simulink library "common_lib"  (R2021b)
settings: Solver=ode45  StartTime=0.0  StopTime=10.0  RelTol=1e-3
undefined symbols (not defined in the file or in its folder): ACCEL_PRE_MULT, C_C1GearNumbers, C_C1GearRatios, C_Calibration, C_DitherWaveform, C_GearOffset, C_GearRatioIn, C_GearRatioInverseOut, C_GearRatioOut, CLUTCH_INNER_LOOP_UPDATE_RATE, CONSTANT, DEGRADED_MODE_SIZE, Dem_EventStatusType, DiscIntNeverNeededParam, F_FAULT_ENUM, F_NOFAULT, F_OUTOFRANGE, F_RATELIMIT, FALSE, FMI14_SPECIAL_INSTRUCTIONS, FMI20_DATA_DRIFTED_HIGH, FMI21_DATA_DRIFTED_LOW, FMI29_RESERVED_FOR_SAE_ASSIGNMENT, FMI30_RESERVED_FOR_SAE_ASSIGNMENT, FMI31_CONDITION_EXISTS, FMI32_NO_FAULT, IC, k_accel, k_mean, LVDCU_OORH_FaultCntThd_C, MAX_UINT32, MEAN_PRE_MULT, NTriggers, QLTY_SIGNAL_FAILED, QLTY_SIGNAL_FULLY_FUNCTION, QLTY_SIGNAL_SUBSTITUTED_BY_1ST_CHOICE, QLTY_SIGNAL_SUBSTITUTED_BY_2ND_CHOICE, QLTY_SIGNAL_SUBSTITUTED_BY_3RD_CHOICE, QLTY_SIGNAL_SUBSTITUTED_BY_4TH_CHOICE, SAMPLE_TIME_100_mSec, SAMPLE_TIME_100_uSec, simin, T_TestPoint, TF_FALSE, TF_TRUE, TimeStep, TRUE, WORKSPACE_UPDATE_RATE, ZERO, Zero
libraries: $bdroot x120, simulink x27, simulink_extras x4, MBD_EPS_Local_Blockset x4
(part 3 of 10)

== system common_lib/SCond ==
  note: Signal Conditioning
  Gain and Offset (in) : Subsystem  mask(CL Gain And Offset (in)){DataType=Single}
      mask prompts: DataType "Output Data Type"
      mask help:
      | Gain/Offset with data type coercion
      |
      | NgEK, Inc.
      mask init:
      | h=gcb;
      | 
      | set_param([h '/InputConversion'], 'DataType','single');
      | set_param([h '/InputConversion1'], 'DataType','single');
      | set_param([h '/InputConversion2'], 'DataType','single');
      | 
      | switch DataType
      |   case (1)
      |       set_param([h '/OutputConversion'], 'DataType','int8');
      |  case (2)
      |       set_param([h '/OutputConversion'], 'DataType','uint8');
      |    case (3)
      |       set_param([h '/OutputConversion'], 'DataType','int16');
      |  case (4)
      |      set_param([h '/OutputConversion'], 'DataType','uint16');
      |   case (5)
      |         set_param([h '/OutputConversion'], 'DataType','single');
      |    case (6)
      |         set_param([h '/InputConversion'], 'DataType','double');
      |         set_param([h '/InputConversion1'], 'DataType','double');
      |         set_param([h '/InputConversion2'], 'DataType','double');
      |      set_param([h '/OutputConversion'], 'DataType','double');    
      |    otherwise
      |      set_param([h '/OutputConversion'], 'DataType','single');
      | end
      mask Help: web(which(['common_lib32.html']))
      mask TypeOptions DataType: Int8 | UInt8 | Int16 | UInt16 | Single | Double
      mask Display:
      | patch([0.35 0.35 0.65 0.65], [0.35 0.65 0.65 0.35], [255/255 127/255 255/255]);
      | disp(['mx-b']);
  Gain and Offset (out) : Subsystem  mask(CL Gain And Offset (out)){DataType=Single}
      mask prompts: DataType "Output Data Type"
      mask help:
      | Gain/Offset with data type coercion
      |
      | NgEK, Inc.
      mask init: same as common_lib/SCond/Gain and Offset (in)
      mask Help: web(which(['common_lib33.html']))
      mask TypeOptions DataType: Int8 | UInt8 | Int16 | UInt16 | Single | Double
      mask Display:
      | patch([0.35 0.35 0.65 0.65], [0.35 0.65 0.65 0.35], [255/255 127/255 255/255]);
      | disp(['(x+b)/m']);
  Membership Function : Subsystem  mask(CL Membership Function){Low=single(10), Peak=single(50), High=single(90), DType=Upper Trapezoid}
      mask prompts: Low "Lower Value"; Peak "Peak Value"; High "Upper Value"; DType "Membership Type"
      mask help:
      | Triangular membership function calculation with an output of 1 at the "Peak" value and dropping off to 0 towards the "Low" and "High" values.  End "trapezoid" membership functions may be specified with the membership "type" pulldown menu.
      |
      | X(1) = Independent Variable
      |
      | Y(1) = Membership Function (0:1)
      |
      | NgEK, Inc.
      mask init:
      | if Peak<Low | Peak>High, disp(['WARNING: Breakpoints Non-Monotonic in <' gcb '>!']), end
      | 
      | switch class(Peak)
      |   case ('double')
      |        Zero      = double( 0.0);
      |          One       = double( 1.0);
      |         if (DType==1)
      |             SlopeLow  = 0.0;
      |           SlopeHigh = 1.0/(Peak-High);
      |         elseif (DType==2)
      |             SlopeLow  = 1.0/(Peak-Low);
      |            SlopeHigh = 1.0/(Peak-High);
      |       else
      |          SlopeLow  = 1.0/(Peak-Low);
      |           SlopeHigh = 0.0;
      |        end;
      |      
      |     case ('single')
      |        Zero      = single( 0.0);
      |          One       = single( 1.0);
      |        if (DType==1)
      |            SlopeLow  = single(0.0);
      |           SlopeHigh = single(1.0/(double(Peak)-double(High)));
      |          elseif (DType==2)
      |            SlopeLow  = single(1.0/(double(Peak)-double(Low)));
      |            SlopeHigh = single(1.0/(double(Peak)-double(High)));
      |       else
      |          SlopeLow  = single(1.0/(double(Peak)-double(Low)));
      |           SlopeHigh = single(0.0);
      |         end;
      | end;
      | 
      | if     (abs(double(SlopeLow))<abs(double(SlopeHigh)))
      |   XPltAxis = [ 0 0.2 0.7 0.8 1.0 ];
      | elseif (abs(double(SlopeHigh))<abs(double(SlopeLow)))
      |  XPltAxis = [ 0 0.2 0.3 0.8 1.0 ];
      | else
      |  XPltAxis = [ 0 0.2 0.5 0.8 1.0 ];
      | end;
      | 
      | if     (DType==1)
      |        YPltAxis = [ 1 1 0 0 0 ];
      | elseif (DType==2)
      |        YPltAxis = [ 0 0 1 0 0 ];
      | else
      |        YPltAxis = [ 0 0 0 1 1 ];
      | end;
      mask Help: web(which(['common_lib36.html']))
      mask TypeOptions DType: Lower Trapezoid | Central Triangle | Upper Trapezoid
      mask Display:
      | patch([.2 .2 .8 .8],[.2 .85 .85 .2],[255/255 127/255 255/255])
      | plot(XPltAxis, YPltAxis);
      | disp(['Low=',num2str(double(Low)),sprintf('\n'),'Peak=',num2str(double(Peak)),sprintf('\n'),'High=',num2str(double(High))])
  Test Override Gain and Offset (in) : Subsystem  mask(CL Gain And Offset (in)){DataType=Single}
      mask prompts: DataType "Output Data Type"
      mask help: Gain/Offset with enabled Gain and Offset option and with Output data type conversion
      mask init: same as common_lib/SCond/Gain and Offset (in)
      mask TypeOptions DataType: Int8 | UInt8 | Int16 | UInt16 | Single | Double
      mask Display:
      | patch([0.3 0.3 0.7 0.7], [0.35 0.65 0.65 0.35], [255/255 127/255 255/255])
      | disp(['Y=mX+b\nTest Override'])
  ramp to zero : Subsystem  mask(CL Ramp to Zero){DataType=Single}
      mask prompts: DataType "Data Type"
      mask help:
      | Ramp input signal to zero
      |
      | X(1) = Speed
      | X(2) = Limit
      |
      | Y(1) = Factor
      |
      | NgEK, Inc.
      mask init:
      | switch DataType
      |     case (1)
      |        One      = single( 1.0);
      |          MinusOne = single(-1.0);
      |         Zero     = single( 0.0);
      |     case (2)
      |         One      = double( 1.0);
      |          MinusOne = double(-1.0);
      |       Zero     = double( 0.0);
      | end;
      mask Help: web(which(['common_lib34.html']))
      mask TypeOptions DataType: Single | Double
      mask Display:
      | patch([0.3 0.3 0.7 0.7], [0.3 0.7 0.7 0.3], [255/255 127/255 255/255]);
      | disp('ramp to\nzero')

== system common_lib/Signal Conditioning ==
  note: Signal Conditioning
  2nd Order Butterworth Filter : Subsystem  mask{IC=0, TSAMP=0}
      mask prompts: IC "Initial Condition"; TSAMP "Sample Time"
      mask Display:
      | patch([0.35 0.35 0.65 0.65], [0.3 0.7 0.7 0.3], [255/255 127/255 255/255])
      | disp('2nd Order\nButterworth')
      | port_label('input',1,'input')
      | port_label('input',2,'cutoff_freq')
      | port_label('input',3,'reset')
      | port_label('output',1,'output')
  AnalogChecking : Subsystem  TreatAsAtomicUnit=on  mask{TimeStep=[]}
      mask prompts: TimeStep "Time Step"
  DitherSaturation : Subsystem  Description=|
      | This block generates dither using the table given for DitherWaveform at the frequency and amplitude given by the freq_hz and amplitude inputs.  All inputs should be 'single' datatype.  The table should be 'single' data type also.  The block runs at the sample time of the 'in' input.  It generates the correct frequency dither regardless of sample time.
      |                                                                                                                                                                                                                                                                                                                                                                  
      | Since it may not be possible to generate the exact frequency specified in the 'freq_hz' input, the block puts out the actual frequency in the 'realized_frequency' output.
  DitherSaturation1 : Subsystem  Description=|
      | This block generates dither using the table given for DitherWaveform at the frequency and amplitude given by the freq_hz and amplitude inputs.  All inputs should be 'single' datatype.  The table should be 'single' data type also.  The block runs at the sample time of the 'in' input.  It generates the correct frequency dither regardless of sample time.
      |                                                                                                                                                                                                                                                                                                                                                                  
      | Since it may not be possible to generate the exact frequency specified in the 'freq_hz' input, the block puts out the actual frequency in the 'realized_frequency' output.
  HydValveDither : Subsystem  Description=|  mask{DitherWaveform=single(C_DitherWaveform), ts=0}
      | This block generates dither using the table given for DitherWaveform at the frequency and amplitude given by the freq_hz and amplitude inputs.  All inputs should be 'single' datatype.  The table should be 'single' data type also.  The block runs at the sample time of the 'in' input.  It generates the correct frequency dither regardless of sample time.
      |                                                                                                                                                                                                                                                                                                                                                                  
      | Since it may not be possible to generate the exact frequency specified in the 'freq_hz' input, the block puts out the actual frequency in the 'realized_frequency' output.
      mask prompts: DitherWaveform "Dither Waveform"; ts "Sample Time"
  Normalized Variable Tanh Curve : Subsystem  mask{TimeStep=TimeStep}
      mask prompts: TimeStep "Sample Time"
      mask Display:
      | patch([0.3 0.3 0.7 0.7], [0.35 0.65 0.65 0.35], [255/255 127/255 255/255])
      | plot([0:.05:1],(tanh(([0:.05:1]*2*pi)-pi)+1)/2)
      | port_label('input',1,'RampTime')
      | port_label('input',2,'Reset')
      | port_label('output',1,'Out')
  Obsolete Signal Conditioning : Subsystem
      mask Display: disp('Obsolete\nSignal\nConditioning')
  OffsetAndGain : Subsystem  TreatAsAtomicUnit=on  mask(CL_OffsetAndGain){}
      mask help: Gain/Offset
      mask Help: web(which(['common_lib32.html']))
      mask Display:
      | patch([0.3 0.3 0.7 0.7], [0.4 0.6 0.6 0.4], [205/255 205/255 255/255]);
      | disp(['m*(x+b)']);
  SpeedProcess : Subsystem
  Trajectory : Subsystem  mask{TimeStep=TimeStep, wn=single(30), damping=single(.8)}
      mask prompts: TimeStep "Sample Time"; wn "Natural Frequency"
      mask Display:
      | patch([0.325 0.325 0.675 0.675], [0.35 0.65 0.65 0.35], [255/255 127/255 255/255])
      | disp('Trajectory')
      | port_label('input',1,'In')
      | port_label('input',2,'MaxAccel')
      | port_label('input',3,'MinAccel')
      | port_label('input',4,'MaxJerk')
      | port_label('input',5,'MinJerk')
      | port_label('input',6,'Reset')
      | port_label('output',1,'Out')
  Variable Tanh Curve : Subsystem  mask{TimeStep=TimeStep}
      mask prompts: TimeStep "Sample Time"
      mask Display:
      | patch([0.3 0.3 0.7 0.7], [0.35 0.65 0.65 0.35], [255/255 127/255 255/255])
      | plot([0:.05:1],(tanh(([0:.05:1]*2*pi)-pi)+1)/2)
      | port_label('input',1,'StartValue')
      | port_label('input',2,'FinalValue')
      | port_label('input',3,'RampTime')
      | port_label('input',4,'Reset')
      | port_label('output',1,'Out')
      | port_label('output',2,'RampComplete')

== system common_lib/Signal Generators ==
  note: Signal Generators
  Clu_2_1_3_1_1_1_TestSignalBuilder : Subsystem
  CustomProfileGenerator : Subsystem  mask{TimeStep=single(0.002)}
      mask prompts: TimeStep "Time Step"
  Signal Generator Components : Subsystem
      mask Display: disp('Signal\nGenerators\nComponents')
  SquareTriangleWaveDither : Subsystem  mask{TimeStep=single(0.002)}
      mask prompts: TimeStep "Time Step"
  SquareTriangleWaveDitherPWM : Subsystem  mask{TimeStep=single(0.002)}
      mask prompts: TimeStep "Time Step"
  SquareTriangleWaveGenerator_Advanced : Subsystem  mask{TimeStep=0}
      mask prompts: TimeStep "Time Step"
  SquareTriangleWaveGenerator_Basic : Subsystem  mask{TimeStep=0}
      mask prompts: TimeStep "Time Step"

== system common_lib/Signal Routing ==
  note: Signal Routing
  Overwrite : Subsystem  mask{VarName=VariableName, OverwriteEnable=off, OverwriteValue=0}
      mask prompts: VarName "Name"; OverwriteEnable "Overwrite ?"; OverwriteValue "Value"
      mask init:
      | enabled = strncmpi(get_param(gcb, 'OverwriteEnable'), 'on', 2);
      | 
      | if (enabled)
      |     dispname = char(get_param(gcb, 'OverwriteValue'));
      | else
      |     dispname = char('No Overwrite');
      | end
      | 
      | dispname = [VarName '\n' dispname];
      | 
      | %
      | % Change the name of the constants to match the VarName
      | %
      | rtblockname = char(find_system(gcb, 'LookUnderMasks', 'all', 'FollowLinks', 'on', 'BlockType', 'Constant'));
      | 
      | % The first constant should be the overwrite enable
      | set_param(deblank(rtblockname(1,:)), 'Name', strcat('xPCOE_', VarName));
      | 
      | % The second constant should be the overwrite value
      | set_param(deblank(rtblockname(2,:)), 'Name', strcat('xPCOV_', VarName));
      mask Display: disp(dispname)
  Vector to Bus : Subsystem  mask(Vector To Bus){BOName=BO_}
      mask prompts: BOName "Bus Object Name (Must be in workspace)"
      mask help:
      | This block takes in a vector and adds the signal names specified in the bus
      | object.  The output is a bus.
      |
      | In the present state of development this block only works for 8 input elements.
      mask init:
      | % Set the number of signals in the input mux.  This should really come from
      | % the dialog box. 
      | NumInputs = 8;
      | 
      | % Get the name of the bus object
      | BOName = get_param(gcb, 'BOName');
      | 
      | % If this workspace var is not of type Simulink.Bus there is a problem
      | a = evalin('base', ['whos(''' BOName ''')']);
      | 
      | if (length(a)==0) 
      |     error('The dialog must specify a valid Simulink.Bus')
      | end
      | if (strcmp(a.class, 'Simulink.Bus')==0)
      |     error('The dialog must specify a valid Simulink.Bus')
      | end
      | 
      | % Find the number of elements in the bus object
      | BONumelm = evalin('base', ['length(' BOName '.Elements)']);
      | 
      | % Get the names from the bus object
      | for x=1:BONumelm
      |     SigNames{x} = evalin('base', [BOName '.Elements(' sprintf('%i',x) ').Name']);
      | end
      | 
      | % Find the bus creator
      | BusCreator = char(find_system(gcb, 'LookUnderMasks', 'all', 'FollowLinks', 'on', 'BlockType', 'BusCreator'));
      | p = get_param(BusCreator, 'PortHandles');
      | l = get_param(p.Inport, 'Line');
      | 
      | % Assign the names to the signals going into the bus creator
      | for x=1:NumInputs
      |     if (x<=BONumelm)
      |        set_param(l{x}, 'Name', SigNames{x});
      |     else
      |        set_param(l{x}, 'Name', sprintf('Signal%i', x));
      |     end
      | end
      mask Display: disp(BOName)

== system common_lib/Slink ==
  note: Simulink Enhancements
  Dead : Subsystem  mask(CL Variable Deadband){DataType=Single}
      mask prompts: DataType "Data Type"
      mask help:
      | Deadband with smooth output transition from deadband region.
      |
      | X(1) = input
      | X(2) = deadband
      |
      | Y(1) = output
      | NgEK, Inc.
      mask init:
      | switch DataType
      |     case (1)
      |        Zero     = double( 0.0);
      |          MinusOne = double(-1.0);
      |     case (2)
      |          Zero     = single( 0.0);
      |       MinusOne = single(-1.0);
      |    case (3)
      |        Zero     = int8( 0.0);
      |         MinusOne = int8(-1.0);
      |     case (4)
      |        Zero     = int16( 0.0);
      |       MinusOne = int16(-1.0);
      |     case (5)
      |          Zero     = int32( 0.0);
      |          MinusOne = int32(-1.0);
      | end;
      mask Help: web(which(['common_lib35.html']))
      mask TypeOptions DataType: Double | Single | Int8 | Int16 | Int32
      mask Display:
      | patch([0.3 0.3 0.7 0.7], [0.35 0.65 0.65 0.35], [255/255 127/255 255/255])
      | 
      | plot([0 1],[0.5 0.5], [0.5 0.5],[0 1], [0.1 0.35],[0.1 0.5], [0.65 0.9],[0.5 0.9])
  Hysteresis : Subsystem  mask(CL Hysteresis){IC=[]}
      mask prompts: IC "Initial Condition"
      mask help:
      | Hysteresis block
      |
      | X(1) = Input
      | X(2) = Deadband Width
      |
      | Y(1) = Output
      | NgEK, Inc.
      mask init:
      | switch class(IC)
      |    case ('double')
      |         MinusOne = double(-1.0);
      |  case ('single')
      |        MinusOne = single(-1.0);
      |  case ('int8')
      |       MinusOne = int8(-1.0);
      |     case ('int16')
      |       MinusOne = int16(-1.0);
      |     case ('int32')
      |          MinusOne = int32(-1.0);
      | end;
      mask Help: web(which(['common_lib42.html']))
      mask Display:
      | patch([0.3 0.3 0.7 0.7], [0.35 0.65 0.65 0.35], [255/255 127/255 255/255])
      | 
      | plot([0 .6 .75 1],[.25 .25 .75 .75], [.25 .4 .75],[.25 .75 .75], [.4 .5 .4],[.35 .25 .15], [.6 .5 .6],[.85 .75 .65])
  Relay : Subsystem  mask(CL Relay){init=[]}
      mask prompts: init "Initiailization State"
      mask help:
      | Relay block
      |
      | X(1) = Input
      | X(2) = Upper Threshold
      | X(3) = Lower Threshold
      | X(4) = Upper Value
      | X(5) = Lower Value
      |
      | Y(1) = output
      | NgEK, Inc.
      mask Help: web(which(['common_lib41.html']))
      mask Display:
      | patch([0.3 0.3 0.7 0.7], [0.35 0.65 0.65 0.35], [255/255 127/255 255/255])
      | 
      | plot([0 .75 .75 1],[.25 .25 .75 .75], [.25 .25 .75],[.25 .75 .75], [.4 .5 .4],[.35 .25 .15], [.6 .5 .6],[.85 .75 .65])
  Relay_1 : Subsystem  mask(CL Relay){}
      mask help:
      | Relay block
      |
      | X(1) = Input
      | X(2) = hysterisis
      | X(3) = Ending Point
      | Y(1) = output
      | NgEK, Inc.
      mask Help: web(which(['common_lib41.html']))
      mask Display:
      | patch([0.3 0.3 0.7 0.7], [0.35 0.65 0.65 0.35], [255/255 127/255 255/255])
      | 
      | plot([0 .75 .75 1],[.25 .25 .75 .75], [.25 .25 .75],[.25 .75 .75], [.4 .5 .4],[.35 .25 .15])
      | 
      | port_label('input', 1, 'Input')
      | port_label('input', 2, 'dead band')
      | port_label('input', 3, 'B')
      | port_label('output', 1, 'out')
  Sat : Subsystem  mask(CL Variable Saturation){}
      mask help:
      | Variable saturation block
      |
      | X(1) = input
      | X(2) = upper limit
      | X(3) = lower limit
      |
      | Y(1) = output
      | NgEK, Inc.
      mask Help: web(which(['common_lib37.html']))
      mask Display:
      | patch([0.3 0.3 0.7 0.7], [0.35 0.65 0.65 0.35], [255/255 127/255 255/255])
      | 
      | plot([0 1],[0.5 0.5],[0.5 0.5],[0 1],[0 0.25 0.75 1],[0 0 1 1])
  Three Value Threshold : Subsystem  mask(CL ThreeValuedThreshold){}
      mask help:
      | Relay block
      |
      | X(1) = Input
      | X(2) = Upper Threshold
      | X(3) = Lower Threshold
      | X(4) = Upper Value
      | X(5) = Between Value
      | X(6) = Lower Value
      |
      | Y(1) = output
      | NgEK, Inc.
      mask Help:
      | Relay block
      | 
      | X(1) = Input
      | X(2) = Upper Threshold
      | X(3) = Lower Threshold
      | X(4) = Upper Value
      | X(5) = Between Value
      | X(6) = Lower Value
      | 
      | Y(1) = output
      | NgEK, Inc.
      mask Display:
      | patch([0.3 0.3 0.7 0.7], [0.35 0.65 0.65 0.35], [255/255 127/255 255/255])
      | 
      | plot([0 0.25 0.25 0.75 0.75 1],[0.25 0.25 0.5 0.5 0.75 0.75]);
      | 
      | %plot([0 .75 .75 1],[.25 .25 .75 .75], [.25 .25 .75],[.25 .75 .75], [.4 .5 .4],[.35 .25 .15], [.6 .5 .6],[.85 .75 .65])
  Variable Rate Limiter : Subsystem  mask(CL Variable Rate Limiter){TimeStep=, ic=}
      mask prompts: TimeStep "Time Step"; ic "Initial Condition"
      mask help:
      | Variable rate limiter block
      |
      | X(1) = input
      | X(2) = rise rate
      | X(3) = fall rate
      |
      | Y(1) = output
      | NgEK, Inc.
      mask Help: web(which(['common_lib38.html']))
      mask Display:
      | patch([0.3 0.3 0.7 0.7], [0.35 0.65 0.65 0.35], [255/255 127/255 255/255])
      | 
      | plot([0 1],[0.5 0.5],[0.5 0.5],[0 1],[0 1],[0 1],[0.7 0.8 0.8],[0.8 0.8 0.7], [0.2 0.2 0.3],[0.3 0.2 0.2])
  Variable Rate Limiter w IC : Subsystem  mask(CL Variable Rate Limiter with Initial Condition){TimeStep=, ic=}
      mask prompts: TimeStep "Time Step"; ic "Initial Condition"
      mask help:
      | Variable rate limiter block with Initial Condiiton
      |
      | X(1) = input
      | X(2) = rise rate
      | X(3) = fall rate
      | X(4) = initial condition
      | X(5) = reset?
      |
      | Y(1) = output
      | NgEK, Inc.
      mask Help: web(which(['common_lib39.html']))
      mask Display:
      | patch([0.3 0.3 0.7 0.7], [0.35 0.65 0.65 0.35], [255/255 127/255 255/255])
      | 
      | plot([0 1],[0.5 0.5],[0.5 0.5],[0 1],[0 1],[0 1],[0.7 0.8 0.8],[0.8 0.8 0.7], [0.2 0.2 0.3],[0.3 0.2 0.2])
  Variable Rate Limiter w IC and Sat : Subsystem  mask(CL Variable Rate Limiter with IC and Saturation){TimeStep=, ic=}
      mask prompts: TimeStep "Time Step"; ic "Initial Condition"
      mask help:
      | Variable rate limiter block with Initial Condition and Saturation
      |
      | X(1) = input
      | X(2) = rise rate
      | X(3) = fall rate
      | X(4) = upper limit
      | X(5) = lower limit
      | X(6) = initial condition
      | X(7) = reset?
      |
      | Y(1) = output
      | NgEK, Inc.
      mask Help: web(which(['common_lib40.html']))
      mask Display:
      | patch([0.3 0.3 0.7 0.7], [0.35 0.65 0.65 0.35], [255/255 127/255 255/255])
      | 
      | plot([0 1],[0.5 0.5],[0.5 0.5],[0 1],[0 0.25 0.75 1],[0 0 1 1],[0.3 0.3 0.45],[0.25 0.1 0.2],[0.55 0.7 0.75],[0.8 0.9 0.78])

== system common_lib/Tbl ==
  note: Tables
  2D Lookup : Subsystem  TreatAsAtomicUnit=on  RTWFcnName=VARTABLE  mask(CL 2D Table Lookup){Mode=Linear Interpolation}
      mask prompts: Mode "Interpolation Mode"
      mask help:
      | 2D Table lookup with explicit axis inputs
      |
      | X(1) = Independent variable
      | X(2) = X axis vector
      | X(3) = Y axis vector
      |
      | Y(1) = output
      |
      | Interpolation mode is selected via the mask:
      |
      | Ceiling Interpolation: rounds up in the positive direction
      | Floor Interpolation: rounds down in the negative direction
      | Nearest (Neighbor) Interpolation: rounds to the closest representable number
      | Linear Interpolation: Interpolates data by assuming data varies linearly between points
      |
      | NgEK, Inc.
      settings: RTWFcnNameOpts=User specified  RTWFileNameOpts=Use function name
      mask Help: web(which(['common_lib45.html']))
      mask TypeOptions Mode: Linear Interpolation | Nearest Neighbor | Floor | Ceiling
      mask Display:
      | patch([0.3 0.3 0.7 0.7], [0.35 0.65 0.65 0.35], [255/255 127/255 255/255])
      | 
      | plot([0.2 0.2],[0.2 0.8],[0.2 0.8],[0.2 0.2],linspace(0.2,0.8,10),0.2+0.8*linspace(0.2,0.8,10).^2)
  Direct Look-Up Table (n-D) : LookupNDDirect
      settings: AttributesFormatString=%<mxTable>
  Interpolator : Subsystem  mask(CL Interpolation){DType=Double}
      mask prompts: DType "Data Type"
      mask help:
      | 1D Interpolation Block
      |
      | X(1) = value at 1
      | X(2) = value at 0
      | X(3) = interpolation value
      |
      | Y(1) = output
      | NgEK, Inc.
      mask init:
      | switch DType
      |    case (1)
      |       set_param([gcb '/XY Interpolator'],'DType','double');
      |        Zero = double(0.0);
      |          One  = double(1.0);
      |     case (2)
      |        set_param([gcb '/XY Interpolator'],'DType','single');
      |         Zero = single(0.0);
      |        One  = single(1.0);
      | end;
      mask Help: web(which(['common_lib43.html']))
      mask TypeOptions DType: Double | Single
      mask Display:
      | patch([0.3 0.3 0.7 0.7], [0.35 0.65 0.65 0.35], [255/255 127/255 255/255])
      | 
      | plot([.2 .9],[0.5 0.5],[0.2 0.3 0.8 .9],[.25 .25 .75 .75])
      | 
      | port_label('input', 1, '1')
      | port_label('input', 2, '0')
      | port_label('input', 3, 'interp')
  Look-Up Table : Lookup  InputValues=[-5:5]  Table=tanh([-5:5])  LookUpMeth=Interpolation-Use End Values
      settings: AttributesFormatString=%<OutputValues>
  Look-Up Table (2-D) : Lookup2D  RowIndex=[1:3]  ColumnIndex=[1:3]  Table=[4 5 6;16 19 20;10 18 23]  LookUpMeth=Interpolation-Use End Values
      settings: AttributesFormatString=%<OutputValues>
  XY Interpolator : Subsystem  TreatAsAtomicUnit=on  RTWFcnName=XYINT  mask(CL XY Interpolation){DType=single}
      mask prompts: DType "Data Type"
      mask help:
      | 2D Interpolation Block
      |
      | X(1) = output value at 1
      | X(2) = output value at 0
      | X(3) = input value corresponding to 1
      | X(4) = input value corresponding to 0
      | X(5) = input value
      |
      | Y(1) = output
      | NgEK, Inc.
      mask init:
      | switch DType
      |    case (1)
      |       set_param([gcb '/Interp'],...
      |          'FunctionName','xyinterp_f64_wrap',...
      |           'SFunctionModules','xyinterp_f64');
      | %        Zero = double(0.0);
      | %          One  = double(1.0);
      | %        Tol  = double(1e-6);
      |     case (2)
      |        set_param([gcb '/Interp'],...
      |           'FunctionName','xyinterp_f32_wrap',...
      |           'SFunctionModules','xyinterp_f32');
      | %        Zero = single(0.0);
      | %        One  = single(1.0);
      | %         Tol  = single(1e-6);
      | end;
      | % strDType = get_param(gcb,'DType');
      | % set_param([gcb '/DTC'],'OutDataTypeStr',strDType);
      | % set_param([gcb '/DTC1'],'OutDataTypeStr',strDType);
      | % set_param([gcb '/DTC2'],'OutDataTypeStr',strDType);
      | % set_param([gcb '/DTC3'],'OutDataTypeStr',strDType);
      | % set_param([gcb '/DTC4'],'OutDataTypeStr',strDType);
      settings: RTWFcnNameOpts=User specified  RTWFileNameOpts=Use function name
      mask Help: web(which(['common_lib44.html']))
      mask TypeOptions DType: double | single
      mask Display:
      | patch([0.3 0.3 0.7 0.7], [0.35 0.65 0.65 0.35], [255/255 127/255 255/255])
      | 
      | plot([.2 .9],[0.5 0.5],[0.2 0.3 0.8 .9],[.25 .25 .75 .75])
      | 
      | port_label('input', 1, 'Y_1')
      | port_label('input', 2, 'Y_0')
      | port_label('input', 3, 'X_1')
      | port_label('input', 4, 'X_0')
      | port_label('input', 5, 'X')
  XY Interpolator1 : Subsystem  TreatAsAtomicUnit=on  RTWFcnName=XYINT  mask(CL XY Interpolation){DType=single}
      mask prompts: DType "Data Type"
      mask help:
      | 2D Interpolation Block
      |
      | X(1) = output value at 1
      | X(2) = output value at 0
      | X(3) = input value corresponding to 1
      | X(4) = input value corresponding to 0
      | X(5) = input value
      |
      | Y(1) = output
      | NgEK, Inc.
      mask init:
      | switch DType
      |    case (1)
      |        Zero = double(0.0);
      |          One  = double(1.0);
      |        Tol  = double(1e-6);
      |     case (2)
      |        Zero = single(0.0);
      |        One  = single(1.0);
      |         Tol  = single(1e-6);
      | end;
      | strDType = get_param(gcb,'DType');
      | set_param([gcb '/DTC'],'OutDataTypeStr',strDType);
      | set_param([gcb '/DTC1'],'OutDataTypeStr',strDType);
      | set_param([gcb '/DTC2'],'OutDataTypeStr',strDType);
      | set_param([gcb '/DTC3'],'OutDataTypeStr',strDType);
      | set_param([gcb '/DTC4'],'OutDataTypeStr',strDType);
      settings: RTWSystemCode=Inline  RTWFcnNameOpts=User specified  RTWFileNameOpts=Use function name
      mask Help: web(which(['common_lib44.html']))
      mask TypeOptions DType: double | single
      mask Display:
      | patch([0.3 0.3 0.7 0.7], [0.35 0.65 0.65 0.35], [255/255 127/255 255/255])
      | 
      | plot([.2 .9],[0.5 0.5],[0.2 0.3 0.8 .9],[.25 .25 .75 .75])
      | 
      | port_label('input', 1, 'Y_1')
      | port_label('input', 2, 'Y_0')
      | port_label('input', 3, 'X_1')
      | port_label('input', 4, 'X_0')
      | port_label('input', 5, 'X')

== system common_lib/Timers ==
  note: Timers
  Timer : Subsystem  mask{TimeStep=0}
      mask prompts: TimeStep "Time Step (double)"
      mask help:
      | This block outputs a boolean true when In has been true
      | for at least the TiggerTime time.

== system common_lib/Approved Simulink/Basic IO ==
  note: HWin/ HWout
  note: Product Test
  note: Data Monitor, VPA, SnapShot
  Inport : Inport
  C_Calibration : $bdroot/IO/Calibration with Pretty Print Value  CalValue=C_Calibration  scaling=None
  Constant : Constant  Value=CONSTANT  SampleTime=-1
  DRDataStoreRead : DataStoreRead  DataStoreName=DataStoreRead  SampleTime=0  IndexOptions=Index vector (dialog)  Indices=1  OutputSizes=1
  DRDataStoreRead1 : DataStoreRead  DataStoreName=PT_ProductTest_Read  SampleTime=0  IndexOptions=Index vector (dialog)  Indices=1  OutputSizes=1
  DRDataStoreRead2 : DataStoreRead  DataStoreName=DM_DataMonitor_Read  SampleTime=0  IndexOptions=Index vector (dialog)  Indices=1  OutputSizes=1
  DSDataStoreMemory : DataStoreMemory  DataStoreName=DataStoreMemory  ShowAdditionalParam=off
  DSDataStoreMemory1 : DataStoreMemory  DataStoreName=PT_ProductTest_Memory  ShowAdditionalParam=off
  DSDataStoreMemory2 : DataStoreMemory  DataStoreName=DM_DataMonitor  ShowAdditionalParam=off
  DWDataStoreWrite : DataStoreWrite  DataStoreName=DataStoreWrite  IndexOptions=Index vector (dialog)  Indices=1  OutputSizes=1
  DWDataStoreWrite1 : DataStoreWrite  DataStoreName=DataStoreWrite  IndexOptions=Index vector (dialog)  Indices=1  OutputSizes=1
  DWDataStoreWrite2 : DataStoreWrite  DataStoreName=DM_DataMonitor_Write  IndexOptions=Index vector (dialog)  Indices=1  OutputSizes=1
  Ground : Ground
  M_MonitorParameter : ToWorkspace  VariableName=MonitorParameter  SampleTime=WORKSPACE_UPDATE_RATE
      settings: Decimation=WORKSPACE_DECIMATION
  M_MonitorParameter1 : Subsystem  mask{work=ToWorkspace}
      mask prompts: work "Variable Name"
      mask init:
      | set_param([gcb,'/towork'],'VariableName',work);
      | a = get_param([gcb '/Input'],'LineHandles');
      | set(a.Outport,'Name',work)
      mask Display:
      | patch([.01 .01 .99 .99],[.01 .99 .99 .01],[0 .8 0])
      | disp(work)
  T_TestPoint : Constant  Value=T_TestPoint  SampleTime=-1
  Terminator : Terminator
  To xPC Scope1 : Subsystem  mask(To Workspace Simulation){UserName=, SampleRate=-1, Prio=Low, NameFromSignal=on}
      mask prompts: UserName "Name"; SampleRate "Sample Rate"; Prio "Priority"; NameFromSignal "Name From Signal"
      mask help:
      | "Green Blocks" will record signals during simulation. The Name is now
      | required to come from the signal name so the "Name From Signal" box should
      | be checked. Please select the appropriate Priority Level to ensure optimal
      | simulation runtime and resource use.
      |
      | High - Will ALWAYS record. Choose this if it is a critical signal that
      |        everyone would benefit from having.
      |
      | Med  - A signal that is important to a particular subsystem for testing
      |        purposes. If testing that subsystem you will likely desire this
      |        signal
      |
      | Low  - For debug purposes within a subsystem. This is for obtaining maximum
      |        information in a subsystem to understand every step of logic during
      |        simulation
      mask init:
      | myPrio = 0;
      | sigName = '';
      | 
      | switch (Prio)
      |     case 'Low'
      |         myPrio = 3;
      |     case 'Med'
      |         myPrio = 2;
      |     case 'High'
      |         myPrio = 1;
      | end
      | 
      | if NameFromSignal || isempty(UserName)
      |     sigName = get_param(gcb, 'InputSignalNames');   % Get the name of the signal
      |     sigName = regexprep(sigName{1}, '[<> ]', '');
      | else
      |     sigName = UserName;
      | end
      | 
      | if ~isempty(sigName)
      |     if myPrio <= getPriority(char(gcb))
      |         tmLst = find_system(gcb, 'FollowLinks', 'on', 'LookUnderMasks', 'on', 'BlockType', 'Terminator');
      |         if ~isempty(tmLst)
      |             pos = get_param(tmLst{1}, 'Position');
      |             delete_block(tmLst{1});
      |             newPos = [pos(1), pos(2), pos(1) + 85, pos(2) + 20];
      |             add_block('built-in/ToWorkspace', [char(gcb) '/ToWorkspace'], ...
      |                 'Position', newPos, ...
      |                 'VariableName', ['SIMOUT_' char(sigName)], ...
      |                 'SampleTime', '-1', ...
      |                 'SaveFormat', 'Structure With Time', ...
      |                 'MaxDataPoints', 'Inf');
      |         end
      |     else
      |         twsLst = find_system(gcb, 'FollowLinks', 'on', 'LookUnderMasks', 'on', 'BlockType', 'ToWorkspace');
      |         if ~isempty(twsLst)
      |             pos = get_param(twsLst{1}, 'Position');
      |             delete_block(twsLst{1});
      |             newPos = [pos(1), pos(2), pos(1) + 20, pos(2) + 20];
      |             add_block('built-in/Terminator', [char(gcb) '/Terminate'], 'Position', newPos);
      |         end
      |     end
      | end
      mask TypeOptions Prio: Low | Med | High
      mask Display: disp(Prio)
  Outport : Outport  VectorParamsAs1DForOutWhenUnconnected=off

== system common_lib/Approved Simulink/Discrete And Discontinuities ==
  Dead Zone Dynamic : simulink/Discontinuities/Dead Zone Dynamic
      settings: SourceProductBaseCode=SL
  Discrete-Time Integrator : DiscreteIntegrator  ICPrevOutput=DiscIntNeverNeededParam  ICPrevScaledInput=DiscIntNeverNeededParam
  Rate Limiter : RateLimiter  SampleTimeMode=inherited
  Relay : Relay
  Saturation : Saturate
  Saturation Dynamic : simulink/Discontinuities/Saturation Dynamic  OutMin=[]  OutMax=[]  OutDataTypeStr=Inherit: Same as second input  OutDataType=fixdt(1, 16)  OutScaling=2^-10  DoSatur=off
  Unit Delay : UnitDelay  InitialCondition=IC  SampleTime=-1  HasFrameUpgradeWarning=on
      settings: AttributesFormatString=ic=%<X0>
  Zero-Order Hold : ZeroOrderHold

== system common_lib/Approved Simulink/Flip Flops ==
  D Flip-Flop : simulink_extras/Flip Flops/D Flip-Flop
  D Latch : simulink_extras/Flip Flops/D Latch
      settings: SourceProductBaseCode=SL
  J-K Flip-Flop : simulink_extras/Flip Flops/J-K Flip-Flop  initial_condition=0
  S-R Flip-Flop : simulink_extras/Flip Flops/S-R Flip-Flop  initial_condition=0

== system common_lib/Approved Simulink/Grouping ==
  note: Busses are preferred to
      | MUXes except where array definition
      | or linear algebra requires a MUX
  Bus Creator : BusCreator  Inputs=2
  Bus Selector : BusSelector  OutputSignals=signal1,signal2
  Demux : Demux  Outputs=2
  Merge : Merge
  Mux : Mux  Inputs=2
  Selector : Selector  InputPortWidth=3  IndexOptions=Index vector (dialog)  Indices=[1 3]  OutputSizes=1

== system common_lib/Approved Simulink/Math And Logic ==
  Abs : Abs  ZeroCross=off
  Assignment : Assignment  IndexOptions=Index vector (dialog)  Indices=1  OutputSizes=1
  Gain : Gain
  Logical Operator : Logic  Operator=OR  AllPortsSameDT=off
  Math Function : Math  SignedPower=on  SaturateOnIntegerOverflow=on
  MinMax : MinMax  Inputs=2  InputSameDT=on  ZeroCross=off
  Multiport Switch : MultiPortSwitch
  Product1 : Product  OutDataTypeStr=Inherit: Same as first input
  Relational Operator : RelationalOperator  Operator=<=  ZeroCross=off  RndMeth=Nearest
  Sign : Signum
  Sum : Sum  Inputs=|+-
  Switch : Switch  Threshold=0.5  ZeroCross=off

== system common_lib/Approved Simulink/Signal Attributes ==
  Data Type Conversion : DataTypeConversion  RndMeth=Zero
  Rate Transition : RateTransition
  Signal Conversion : SignalConversion  ConversionOutput=Contiguous copy  OverrideOpt=off

== system common_lib/Approved Simulink/SubSys Triggers ==
  Enable : EnablePort  ZeroCross=off
  Trigger : TriggerPort  VariantControl=(inherit)  ZeroCross=off
  Configurable Subsystem : Subsystem
      settings: TemplateBlock=self
  For Iterator Subsystem : Subsystem  TreatAsAtomicUnit=on
  Function-Call Generator : simulink/Ports & Subsystems/Function-Call Generator  sample_time=1  numberOfIterations=1  DisallowWideOutput=off
  If : If
  If Action Subsystem : Subsystem  TreatAsAtomicUnit=on
  Subsystem : Subsystem
  Switch Case : SwitchCase
  While Iterator Subsystem : Subsystem  TreatAsAtomicUnit=on

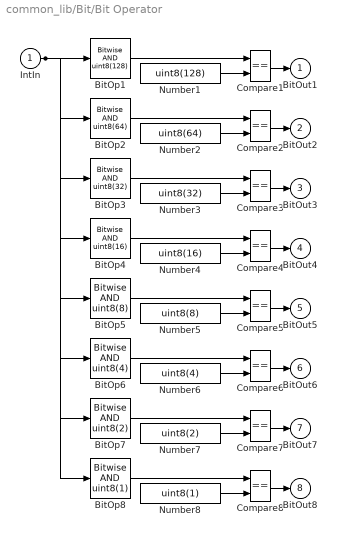
== system common_lib/Bit/Bit Operator ==
  IntIn : Inport
  BitOp1 : simulink/Logic and Bit Operations/Bitwise Operator  logicop=AND  UseBitMask=on  BitMask=uint8(128)  BitMaskRealWorld=Stored Integer
  BitOp2 : simulink/Logic and Bit Operations/Bitwise Operator  logicop=AND  UseBitMask=on  BitMask=uint8(64)  BitMaskRealWorld=Stored Integer
  BitOp3 : simulink/Logic and Bit Operations/Bitwise Operator  logicop=AND  UseBitMask=on  BitMask=uint8(32)  BitMaskRealWorld=Stored Integer
  BitOp4 : simulink/Logic and Bit Operations/Bitwise Operator  logicop=AND  UseBitMask=on  BitMask=uint8(16)  BitMaskRealWorld=Stored Integer
  BitOp5 : simulink/Logic and Bit Operations/Bitwise Operator  logicop=AND  UseBitMask=on  BitMask=uint8(8)  BitMaskRealWorld=Stored Integer
  BitOp6 : simulink/Logic and Bit Operations/Bitwise Operator  logicop=AND  UseBitMask=on  BitMask=uint8(4)  BitMaskRealWorld=Stored Integer
  BitOp7 : simulink/Logic and Bit Operations/Bitwise Operator  logicop=AND  UseBitMask=on  BitMask=uint8(2)  BitMaskRealWorld=Stored Integer
  BitOp8 : simulink/Logic and Bit Operations/Bitwise Operator  logicop=AND  UseBitMask=on  BitMask=uint8(1)  BitMaskRealWorld=Stored Integer
  Compare{1..8} (8 alike) : RelationalOperator  Operator===  RndMeth=Nearest  InputSameDT=on
  Number1 : Constant  Value=uint8(128)
  Number2 : Constant  Value=uint8(64)
  Number3 : Constant  Value=uint8(32)
  Number4 : Constant  Value=uint8(16)
  Number5 : Constant  Value=uint8(8)
  Number6 : Constant  Value=uint8(4)
  Number7 : Constant  Value=uint8(2)
  Number8 : Constant  Value=uint8(1)
  BitOut1 : Outport  VectorParamsAs1DForOutWhenUnconnected=off
  BitOut2 : Outport  Port=2  VectorParamsAs1DForOutWhenUnconnected=off
  BitOut3 : Outport  Port=3  VectorParamsAs1DForOutWhenUnconnected=off
  BitOut4 : Outport  Port=4  VectorParamsAs1DForOutWhenUnconnected=off
  BitOut5 : Outport  Port=5  VectorParamsAs1DForOutWhenUnconnected=off
  BitOut6 : Outport  Port=6  VectorParamsAs1DForOutWhenUnconnected=off
  BitOut7 : Outport  Port=7  VectorParamsAs1DForOutWhenUnconnected=off
  BitOut8 : Outport  Port=8  VectorParamsAs1DForOutWhenUnconnected=off
  wires:
  BitOp1/1 -> Compare1/1
  Number1/1 -> Compare1/2
  Compare1/1 -> BitOut1/1
  IntIn/1 -> BitOp1/1, BitOp2/1, BitOp3/1, BitOp4/1, BitOp5/1, BitOp6/1, BitOp7/1, BitOp8/1
  BitOp2/1 -> Compare2/1
  Number2/1 -> Compare2/2
  Compare2/1 -> BitOut2/1
  BitOp3/1 -> Compare3/1
  Number3/1 -> Compare3/2
  Compare3/1 -> BitOut3/1
  BitOp4/1 -> Compare4/1
  Number4/1 -> Compare4/2
  Compare4/1 -> BitOut4/1
  BitOp5/1 -> Compare5/1
  Number5/1 -> Compare5/2
  Compare5/1 -> BitOut5/1
  BitOp6/1 -> Compare6/1
  Number6/1 -> Compare6/2
  Compare6/1 -> BitOut6/1
  BitOp7/1 -> Compare7/1
  Number7/1 -> Compare7/2
  Compare7/1 -> BitOut7/1
  BitOp8/1 -> Compare8/1
  Number8/1 -> Compare8/2
  Compare8/1 -> BitOut8/1

== system common_lib/Ctrl/DTNA_PIgov ==
  note: During reset, integrator is set to zero
  note: Output - Pterm - Dterm = Iterm for saturation purposes
  note: Detect output saturation
  note: Common Library::Control Structures::PI Governor
  note: pterm
      | limited to output saturation limits
  error : Inport
  p_gain : Inport  Port=2
  i_gain : Inport  Port=3
  ulim : Inport  Port=4
  llim : Inport  Port=5
  reset? : Inport  Port=6  OutDataTypeStr=boolean
  Abs : Abs  ZeroCross=off  OutDataTypeStr=Inherit: Inherit via back propagation
  Constant1 : Constant  Value=MinInt  OutDataTypeStr=Inherit: Inherit via back propagation
  Constant2 : Constant  Value=MaxInt  OutDataTypeStr=Inherit: Inherit via back propagation
  Constant3 : Constant  Value=Zero
  Constant4 : Constant  Value=Zero
  Constant5 : Constant  Value=Tol  OutDataTypeStr=Inherit: Inherit via back propagation
  Integrator : Subsystem  TreatAsAtomicUnit=on  RTWFcnName=INTEGRATOR  mask(CL Integrator){TimeStep=TimeStep, IC=IC}
      mask prompts: TimeStep "Time Step"; IC "Initial Condition"
      mask help:
      | Determine the integral of the input.
      | If reset is true (1), the integrator is set to the reset condition input.
      |
      | X(1) = input
      | X(2) = upper limit
      | X(3) = lower limit
      | X(4) = reset condition
      | X(5) = reset
      |
      | Y(1) = output
      |
      | Time step is entered via mask parameter.
      | Initial condition is entered via mask parameter.
      |
      | NgEK, Inc.
      settings: RTWFcnNameOpts=User specified  RTWFileNameOpts=Use function name
      mask Help: web(which(['common_lib3.html']))
      mask Display:
      | patch([0.3 0.3 0.7 0.7], [0.35 0.65 0.65 0.35], [255/255 127/255 255/255])
      | disp('Integrator')
      | port_label('input', 1, 'input')
      | port_label('input', 2, 'ulim')
      | port_label('input', 3, 'llim')
      | port_label('input', 4, 'reset_cond')
      | port_label('input', 5, 'reset?')
      | port_label('output', 1, 'output')
  Logical Operator : Logic  Operator=OR
  Product1 : Product  InputSameDT=on  OutDataTypeStr=Inherit: Same as first input
  Product2 : Product  InputSameDT=on  OutDataTypeStr=Inherit: Same as first input
  Relational Operator : RelationalOperator  Operator=>  ZeroCross=off  RndMeth=Nearest  InputSameDT=on
  Sat : $bdroot/Slink/Sat
  Sat1 : $bdroot/Slink/Sat
  Sum1 : Sum  Inputs=+-  InputSameDT=on  OutDataTypeStr=Inherit: Same as first input
  Sum2 : Sum  Inputs=+-|  InputSameDT=on  OutDataTypeStr=Inherit: Same as first input
  Sum3 : Sum  InputSameDT=on  OutDataTypeStr=Inherit: Same as first input
  Switch : Switch  Threshold=0.5  ZeroCross=off  InputSameDT=on
  Switch1 : Switch  Threshold=0.5  ZeroCross=off  InputSameDT=on
  Unit Delay1 : UnitDelay  InitialCondition=Zero  SampleTime=-1  HasFrameUpgradeWarning=on
      settings: AttributesFormatString=ic=%<X0>
  Unit Delay2 : UnitDelay  InitialCondition=false  SampleTime=-1  HasFrameUpgradeWarning=on
      settings: AttributesFormatString=ic=%<X0>
  output : Outport  InitialOutput=8.973  VectorParamsAs1DForOutWhenUnconnected=off
  wires:
  Product2/1 -> Integrator/1(input)
  Sum1/1 -> Unit Delay1/1
  Integrator/1(Output) -> Sum3/2
  Switch/1 -> Integrator/4(ic)
  Unit Delay2/1 -> Logical Operator/2
  Logical Operator/1 -> Integrator/5(reset?)
  Constant4/1 -> Switch/1
  i_gain/1 -> Product2/2
  Sat/1 -> Sum2/2, output/1, Sum1/1
  Sum3/1 -> Sum2/1, Sat/1  "Actuator Signal"
  llim/1 -> Sat/3, Sat1/3
  Product1/1 -> Sat1/1, Sum3/1
  p_gain/1 -> Product1/1
  ulim/1 -> Sat/2, Sat1/2
  reset?/1 -> Switch/2, Switch1/2, Logical Operator/1
  Constant1/1 -> Integrator/3(llim)
  Constant2/1 -> Integrator/2(ulim)
  Constant5/1 -> Relational Operator/2
  Abs/1 -> Relational Operator/1
  Relational Operator/1 -> Unit Delay2/1
  Sum2/1 -> Abs/1
  Unit Delay1/1 -> Switch/3
  Sat1/1 -> Sum1/2
  Constant3/1 -> Switch1/1
  error/1 -> Switch1/3
  Switch1/1 -> Product2/1, Product1/2

== system common_lib/Ctrl/Derivative ==
  note: Common Library::Derivative
  input : Inport
  cutoff : Inport  Port=2
  ulim : Inport  Port=3
  llim : Inport  Port=4
  reset? : Inport  Port=5  OutDataTypeStr=boolean
  Data Type Conversion : DataTypeConversion  OutDataTypeStr=boolean
  Data Type Conversion1 : DataTypeConversion  OutDataTypeStr=single
  Data Type Conversion2 : DataTypeConversion  OutDataTypeStr=single
  DerivativeCoreLogic : Subsystem  TreatAsAtomicUnit=on  RTWFcnName=DER
      settings: RTWFcnNameOpts=User specified  RTWFileNameOpts=Use function name
  Gain : Gain  Gain=Ts
  Product1 : Product  Inputs=**  InputSameDT=on  OutDataTypeStr=Inherit: Same as first input
  Signal Conversion : SignalConversion  ConversionOutput=Contiguous copy  OverrideOpt=off
  output : Outport  VectorParamsAs1DForOutWhenUnconnected=off
  wires:
  input/1 -> Product1/1
  cutoff/1 -> Product1/2, Gain/1
  DerivativeCoreLogic/1(output) -> Signal Conversion/1
  reset?/1 -> Data Type Conversion/1
  Gain/1 -> DerivativeCoreLogic/2(cutoff)
  Product1/1 -> DerivativeCoreLogic/1(input)
  ulim/1 -> Data Type Conversion1/1
  llim/1 -> Data Type Conversion2/1
  Data Type Conversion/1 -> DerivativeCoreLogic/3(reset?)
  Data Type Conversion1/1 -> DerivativeCoreLogic/4(ulim)
  Data Type Conversion2/1 -> DerivativeCoreLogic/5(llim)
  Signal Conversion/1 -> output/1

== system common_lib/Ctrl/Dither ==
  note: Filter output waveform to smooth
      | the transitions if necessary.
  note: Keep present output state until
      | number of executions has occured.
      | (initialize to FALSE)
  note: Keep track of number of iterations
      | since last output transition.
      | (initialize to zero)
  note: Calculate number of executions
      | between alternating output.
      | 1/ (2 * TimeStep * frequency)
      | Add in half a frame to roundoff to
      | nearest minor frame boundary
  note: Simple Dither Function
      | Outputs a modified rectangular wave of specified
      | amplitude, frequency and filter constant.
  note: Common Library::Dither
  amplitude : Inport
  frequency : Inport  Port=2
  tau : Inport  Port=3
  Constant1 : Constant  Value=MinusOne
  Constant14 : Constant  Value=int16(1)
  Constant2 : Constant  Value=One
  Constant3 : Constant  Value=Two
  Constant4 : Constant  Value=One
  Constant5 : Constant  Value=lim
  Constant6 : Constant  Value=One
  Constant7 : Constant  Value=int16(1)
  Constant8 : Constant  Value=TimeStep
  Constant9 : Constant  Value=ZeroFive
  Data Type Conversion : DataTypeConversion  OutDataTypeStr=single  RndMeth=Zero
  Data Type Conversion1 : DataTypeConversion  OutDataTypeStr=single
  Fltr : $bdroot/Fltrs/Fltr  TimeStep=TimeStep
  Logical Operator : Logic  Operator=NOT
  MinMax1 : MinMax  Inputs=2  InputSameDT=on  SaturateOnIntegerOverflow=on  ZeroCross=off
  MinMax2 : MinMax  Function=max  Inputs=2  InputSameDT=on  SaturateOnIntegerOverflow=on  ZeroCross=off
  Product1 : Product  Inputs=**  InputSameDT=on  OutDataTypeStr=Inherit: Same as first input
  Product2 : Product  Inputs=***  InputSameDT=on  OutDataTypeStr=Inherit: Same as first input
  Product3 : Product  Inputs=*/  InputSameDT=on  OutDataTypeStr=Inherit: Same as first input
  Relational Operator : RelationalOperator  Operator=<  ZeroCross=off  RndMeth=Nearest  InputSameDT=on
  Sum1 : Sum  Inputs=|++  InputSameDT=on  OutDataTypeStr=Inherit: Same as first input
  Sum3 : Sum  Inputs=++|  InputSameDT=on  OutDataTypeStr=Inherit: Same as first input
  Switch1 : Switch  Threshold=0.5  ZeroCross=off  InputSameDT=on
  Switch2 : Switch  Threshold=0.5  ZeroCross=off  InputSameDT=on
  Switch3 : Switch  Threshold=0.5  ZeroCross=off  InputSameDT=on
  Unit Delay1 : UnitDelay  InitialCondition=int16(0)  SampleTime=-1  HasFrameUpgradeWarning=on
  Unit Delay11 : UnitDelay  InitialCondition=false  SampleTime=-1  HasFrameUpgradeWarning=on
  output : Outport  VectorParamsAs1DForOutWhenUnconnected=off
  wires:
  Constant8/1 -> Data Type Conversion1/1
  Data Type Conversion1/1 -> Product2/1
  Constant9/1 -> Sum1/2
  Sum1/1 -> Relational Operator/2
  Data Type Conversion/1 -> Relational Operator/1
  Relational Operator/1 -> Switch1/2, Switch3/2
  Product3/1 -> Sum1/1
  Logical Operator/1 -> Switch1/3
  Sum3/1 -> Data Type Conversion/1, Switch3/1
  Constant7/1 -> Sum3/1
  Unit Delay1/1 -> Sum3/2
  Constant14/1 -> Switch3/3
  Switch3/1 -> Unit Delay1/1
  Constant3/1 -> Product2/3
  Constant6/1 -> Product3/1
  MinMax2/1 -> Product3/2
  Fltr/1 -> output/1
  Constant5/1 -> MinMax2/2
  MinMax1/1 -> MinMax2/1
  Constant4/1 -> MinMax1/2
  Product2/1 -> MinMax1/1
  frequency/1 -> Product2/2
  amplitude/1 -> Product1/1
  Switch2/1 -> Product1/2
  Constant2/1 -> Switch2/1
  Constant1/1 -> Switch2/3
  Product1/1 -> Fltr/1
  Switch1/1 -> Switch2/2, Unit Delay11/1
  Unit Delay11/1 -> Switch1/1, Logical Operator/1
  tau/1 -> Fltr/2
